simulink model "fault_bus"  (R2014a)
settings: Solver=ode23t  StartTime=0.0  StopTime=1  RelTol=1e-3
settings Model: Creator=Divya M  LastModifiedBy=Divya M

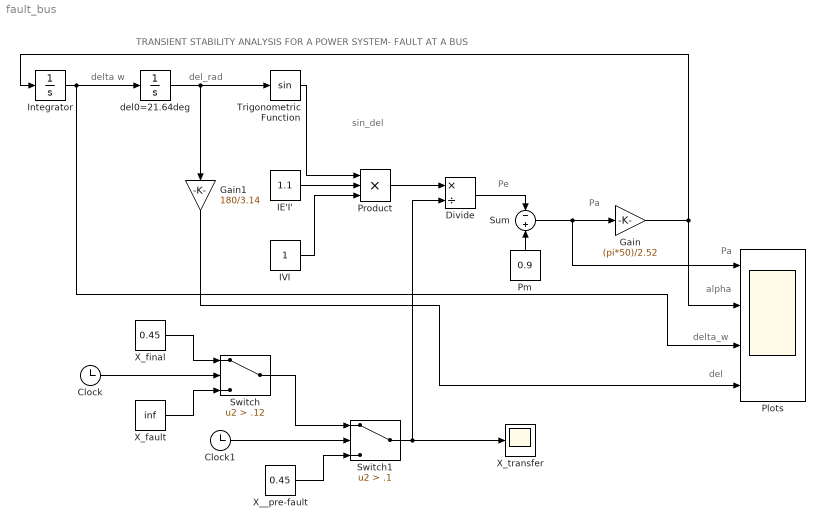
== system fault_bus ==
  note: Pa
  note: Pe
  note: sin_del
  note: del_rad
  note: delta w
  note: TRANSIENT STABILITY ANALYSIS FOR A POWER SYSTEM- FAULT AT A BUS
  note: del
  note: delta_w
  note: alpha
  note: Pa
  Clock : Clock
  Clock1 : Clock
  Divide : Product  Inputs=*/
  Gain : Gain  Gain=(pi*50)/2.52
  Gain1 : Gain  Gain=180/3.14
  IE'I' : Constant  Value=1.1
  IVI : Constant
  Integrator : Integrator
  Plots : Scope  NumInputPorts=4
      settings: YMin=-0.3~-1000~-10~20  YMax=0.3~1000~10~35  SaveName=ScopeData2
  Pm : Constant  Value=0.9
  Product : Product  Inputs=3
  Sum : Sum  Inputs=-+
  Switch : Switch  Criteria=u2 > Threshold  Threshold=.12  ZeroCross=off
  Switch1 : Switch  Criteria=u2 > Threshold  Threshold=.1
  Trigonometric Function : Trigonometry
  X__pre-fault : Constant  Value=0.45
  X_fault : Constant  Value=inf
  X_final : Constant  Value=0.45
  X_transfer : Scope
  del0=21.64deg : Integrator  InitialCondition=(21.64*3.14)/180
  wires:
  Integrator/1 -> Plots/3, del0=21.64deg/1
  del0=21.64deg/1 -> Gain1/1, Trigonometric Function/1
  Trigonometric Function/1 -> Product/1
  IE'I'/1 -> Product/2
  IVI/1 -> Product/3
  Product/1 -> Divide/1
  X_final/1 -> Switch/1
  Clock/1 -> Switch/2
  X_fault/1 -> Switch/3
  Pm/1 -> Sum/2
  Sum/1 -> Plots/1, Gain/1
  Gain/1 -> Plots/2, Integrator/1
  Switch/1 -> Switch1/1
  Clock1/1 -> Switch1/2
  X__pre-fault/1 -> Switch1/3
  Switch1/1 -> X_transfer/1, Divide/2
  Divide/1 -> Sum/1
  Gain1/1 -> Plots/4
